simulink model "Forward_Simulink"  (R2015a)
settings: Solver=ode3  StartTime=0.0  StopTime=tf  FixedStep=t_step  RelTol=1e-3
values from neighbouring files (symbols this model uses):
  Amp = 1    [Forward_Simulation.m]
  C = [Rl/(Rl+RCf),  Rl*RCf/(Rl+RCf)]    [Controller.m]    (also in Controller_ID.m; Controller_ID_Noise.m; Controller_MOD_Hard.m; Controller_MOD_Soft.m)
  C_bulk = 1e-3    (= 0.001)    [Forward_Simulation.m]
  Dmax = 0.366357    [Bridge_Bulk.m]    (also in Controller.m = 0.45; Controller_ID.m = 0.45; Controller_ID_Noise.m = 0.45; Controller_MOD_Hard.m = 0.45)
  F_line = 60    [Forward_Simulation.m]
  F_PWM = 1e5    (= 100000)    [Forward_Simulation.m]
  K = dlqr(alpha*Ad_aug, alpha*Bd_aug, Q1, Q2)    [Controller.m]    (also in Controller_ID.m = [0.033293762099687, 0.032463881530606,      0.00023052612695; Controller_ID_Noise.m = [0.033293762099687, 0.032463881530606,      0.00023052612695; Controller_MOD_Hard.m = [0.033293762099687, 0.032463881530606,      0.00023052612695; Controller_MOD_Soft.m = [0.033293762099687, 0.032463881530606,      0.00023052612695)
  L = 100e-6    (= 0.0001)    [Forward_Design.m]    (also in Forward_Simulation.m; LC_output_filter.m)
  L_leak = 0.45e-6    (= 4.5e-07)    [Forward_Simulation.m]
  Lm = 180e-6    (= 0.00018)    [Forward_Simulation.m]    (also in transformer_design.m = mu_F * N1^2 * Ac * 1e-2 / lm)
  PT = 90    [Forward_Simulation.m]    (also in transformer_design.m = Kfe * Bop^beta * Ac * lm +          rho * MLT * N1^2 * I_RMS)
  r = 2    [Forward_Simulation.m]
  R_load = 1e3    (= 1000)    [Forward_Simulation.m]
  RC = 21e-3    (= 0.021)    [Forward_Design.m]    (also in Forward_Simulation.m = 0.02)
  RC_bulk = 0.03    [Forward_Simulation.m]
  RL = 25e-3    (= 0.025)    [Forward_Design.m]    (also in Forward_Simulation.m)
  Rm = 100    [Forward_Simulation.m]
  RT1 = 0.025    [Forward_Simulation.m]    (also in transformer_design.m = rw_v(pos1) * N1 * MLT)
  RT2 = 0.01    [Forward_Simulation.m]    (also in transformer_design.m = rw_v(pos2) * N2 * MLT)
  T_ctrl = 1e-4    (= 0.0001)    [Forward_Simulation.m]
  t_init = 0.1    [Forward_Simulation.m]
  t_step = Ts / 10    (= 1e-06)    [Controller.m]    (also in Controller_ID.m; Controller_ID_Noise.m; Controller_MOD_Hard.m; Controller_MOD_Soft.m)
  Vp = sqrt(2) * 100    [Bridge_Bulk.m]    (also in Forward_Simulation.m = sqrt(2) * 127)
  VT1rms = 201    [Forward_Simulation.m]
  VT2rms = VT1rms / 1.5    (= 134)    [Forward_Simulation.m]
libraries: powerlib x20, powerlib_meascontrol x1
settings Model: Creator=Marcelo  LastModifiedBy=Marcelo

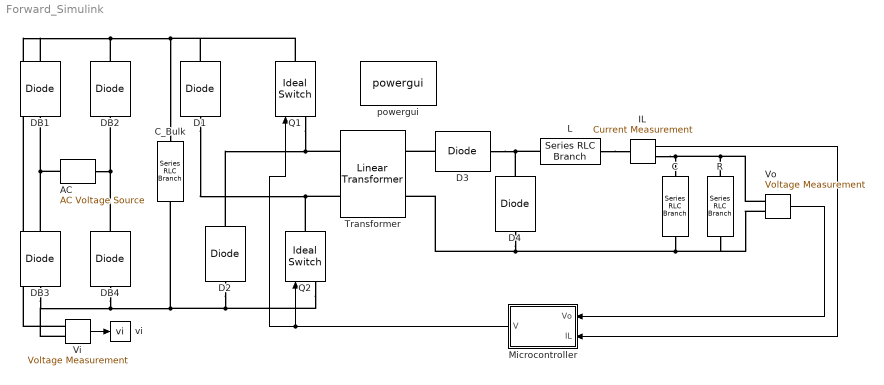
== system Forward_Simulink ==
  AC : powerlib/Electrical Sources/AC Voltage Source  Amplitude=Vp  Phase=0  Frequency=F_line  SampleTime=0  Measurements=None
  C : powerlib/Elements/Series RLC Branch  LConnTagsString=__new0  RConnTagsString=__new0  BranchType=RC  Resistance=RC  Inductance=1e-3  SetiL0=off  InitialCurrent=0  Capacitance=C  Setx0=off  InitialVoltage=0  Measurements=None
  C_Bulk : powerlib/Elements/Series RLC Branch  LConnTagsString=__new0  RConnTagsString=__new0  BranchType=RC  Resistance=RC_bulk  Inductance=1e-3  SetiL0=off  InitialCurrent=0  Capacitance=C_bulk  Setx0=off  InitialVoltage=0  Measurements=None
  D{1..4} (4 alike) : powerlib/Power Electronics/Diode  Ron=Rf  Lon=0  Vf=Vf  IC=0  UseSnubber=off  Rs=1e8  Cs=inf  Measurements=off
  DB{1..4} (4 alike) : powerlib/Power Electronics/Diode  Ron=Rf  Lon=0  Vf=Vf  IC=0  UseSnubber=off  Rs=1e8  Cs=inf  Measurements=off
  IL : powerlib/Measurements/Current Measurement  PhasorSimulation=off  OutputType=Complex  PSBequivalent=0
  L : powerlib/Elements/Series RLC Branch  LConnTagsString=__new0  RConnTagsString=__new0  BranchType=RL  Resistance=RL  Inductance=L  SetiL0=off  InitialCurrent=0  Capacitance=1e-3  Setx0=off  InitialVoltage=0  Measurements=None
  Microcontroller : Subsystem
  Q1 : powerlib/Power Electronics/Ideal Switch  Ron=RDS  Lon=0  IC=0  Rs=1e8  Cs=inf  Measurements=off
  Q2 : powerlib/Power Electronics/Ideal Switch  Ron=RDS  Lon=0  IC=0  Rs=1e8  Cs=inf  Measurements=off
  R : powerlib/Elements/Series RLC Branch  LConnTagsString=__new0  RConnTagsString=__new0  BranchType=R  Resistance=R_load  Inductance=1e-3  SetiL0=off  InitialCurrent=0  Capacitance=1e-3  Setx0=off  InitialVoltage=0  Measurements=None
  Transformer : powerlib/Elements/Linear Transformer  UNITS=SI  NominalPower=[PT, F_PWM]  winding1=[VT1rms, RT1, L_leak]  winding2=[VT2rms, RT2, L_leak]  ThreeWindings=off  winding3=[3.15e+05 0.7938 0.084225]  RmLm=[Rm, Lm]  Measurements=None  DataType=on
  Vi : powerlib/Measurements/Voltage Measurement  PhasorSimulation=off  OutputType=Complex  PSBequivalent=0
  Vo : powerlib/Measurements/Voltage Measurement  PhasorSimulation=off  OutputType=Complex  PSBequivalent=0
  powergui : powerlib/powergui  Priority=1  SimulationMode=Discrete  SolverType=Backward Euler  SampleTime=t_step  frequency=60  SPID=on  DisableSnubberDevices=on  DisableRonSwitches=on  DisableVfSwitches=on  SwTol=0  DisplayEquations=off  Interpol=off  methode=off  Ts=100  FunctionMessages=on  echomessages=off  HookPort=off  EnableUseOfTLC=off  x0status=zero  frequencyindice=60  Pbase=100e6  ErrMax=1e-4  Iterations=50  UnitsV=V  UnitsW=W  buscounter=0  RestoreLinks=warning  ResistiveCurrentMeasurement=off  Frange=[0:2:500]  Ylog=off  Xlog=on  ShowGrid=off  save=off  variable=ZData  structure=0  ZoomFFT=off  StartTime=0.0  cycles=1  DisplayStyle=1  fundamental=60  FreqAxis=off  MaxFrequency=1000  frequencyindicesteady=1  RmsSteady=1  display=off
  vi : ToWorkspace  VariableName=vi  SampleTime=-1
  wires:
  Vi/1 -> vi/1
  Microcontroller/1(V) -> Q2/1, Q1/1
  Vo/1 -> Microcontroller/1(Vo)
  IL/1 -> Microcontroller/2(IL)
  connections:
  Q1/RConn1 -- D1/RConn1 -- Vi/LConn1 -- DB1/RConn1 -- DB2/RConn1 -- C_Bulk/LConn1
  D2/LConn1 -- Q2/LConn1 -- DB3/LConn1 -- Vi/LConn2 -- DB4/LConn1 -- C_Bulk/RConn1
  D3/LConn1 -- Transformer/RConn1
  D3/RConn1 -- L/RConn1 -- D4/RConn1
  C/RConn1 -- Vo/LConn2 -- R/RConn1 -- D4/LConn1 -- Transformer/RConn2
  R/LConn1 -- Vo/LConn1 -- IL/RConn1 -- C/LConn1
  Transformer/LConn1 -- Q1/LConn1 -- D2/RConn1
  Transformer/LConn2 -- Q2/RConn1 -- D1/LConn1
  L/LConn1 -- IL/LConn1
  AC/LConn1 -- DB1/LConn1 -- DB3/RConn1
  AC/RConn1 -- DB4/RConn1 -- DB2/LConn1

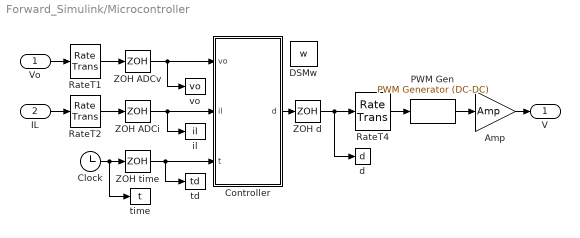
== system Forward_Simulink/Microcontroller ==
  Vo : Inport
  IL : Inport  Port=2
  Amp : Gain  Gain=Amp
  Clock : Clock
  Controller : MATLAB Function  TreatAsAtomicUnit=on  SystemSampleTime=T_ctrl
  DSMw : DataStoreMemory  DataStoreName=w  OutDataTypeStr=double
  PWM Gen : powerlib_meascontrol/Pulse & Signal Generators/PWM Generator (DC-DC)  Fsw=F_PWM  Ts=0
  RateT1 : RateTransition  OutPortSampleTime=T_ctrl
  RateT2 : RateTransition  OutPortSampleTime=T_ctrl
  RateT4 : RateTransition
  ZOH ADCi : ZeroOrderHold  SampleTime=T_ctrl
  ZOH ADCv : ZeroOrderHold  SampleTime=T_ctrl
  ZOH d : ZeroOrderHold  SampleTime=T_ctrl
  ZOH time : ZeroOrderHold  SampleTime=T_ctrl
  d : ToWorkspace  VariableName=d  SampleTime=-1
  il : ToWorkspace  VariableName=il  SampleTime=-1
  td : ToWorkspace  VariableName=td  SampleTime=-1
  time : ToWorkspace  VariableName=t  SampleTime=-1
  vo : ToWorkspace  VariableName=vo  SampleTime=-1
  V : Outport
  wires:
  Clock/1 -> time/1, ZOH time/1
  ZOH ADCv/1 -> vo/1, Controller/1(vo)
  Vo/1 -> RateT1/1
  IL/1 -> RateT2/1
  ZOH ADCi/1 -> Controller/2(il), il/1
  Controller/1(d) -> ZOH d/1
  ZOH d/1 -> d/1, RateT4/1
  PWM Gen/1 -> Amp/1
  Amp/1 -> V/1
  ZOH time/1 -> td/1, Controller/3(t)
  RateT4/1 -> PWM Gen/1
  RateT2/1 -> ZOH ADCi/1
  RateT1/1 -> ZOH ADCv/1

== matlab function Forward_Simulink/Microcontroller/Controller ==
  data: vo input; il input; d output; t input; K parameter; w data_store_memory; r parameter; Dmax parameter; t_init parameter; RC parameter
function d = fcn(vo, il, t, K, r, Dmax, t_init, RC)
global w;
if t > t_init
    y = vo;
    w = w + y - r;
    vc = vo - RC * il;
    d = - K * [vc; il; w];
    if d < 0
        d = 0;
    elseif d > Dmax
        d = Dmax;
    end
else
    d = 0;
end
